simulink model "pipeadc_3b_model"  (R2024b)
settings: Solver=ode4  StartTime=0.0  StopTime=tstop  FixedStep=tstep  RelTol=1e-3
values from neighbouring files (symbols this model uses):
  amplitude = Vref    (= 1.5)    [pipeadc_3b.m]
  fsig = 1e3    (= 1000)    [pipeadc_3b.m]
  offset = 0    [pipeadc_3b.m]
  Vref = (Vrefp-Vrefn)    (= 1.5)    [pipeadc_3b.m]
libraries: simulink_extras x5
settings Model: Creator=koefinger  LastModifiedBy=koefinger

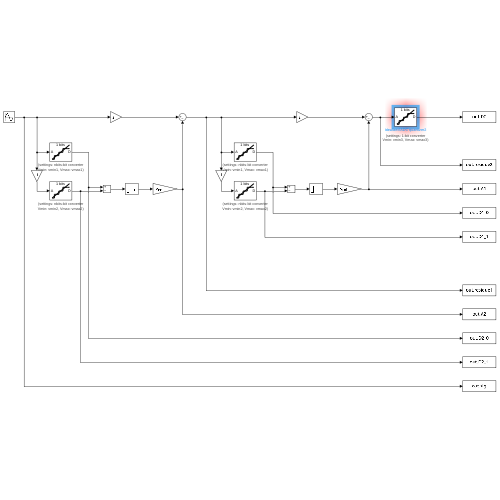
[thumbnail: Simulink's stored preview of the top-level diagram]
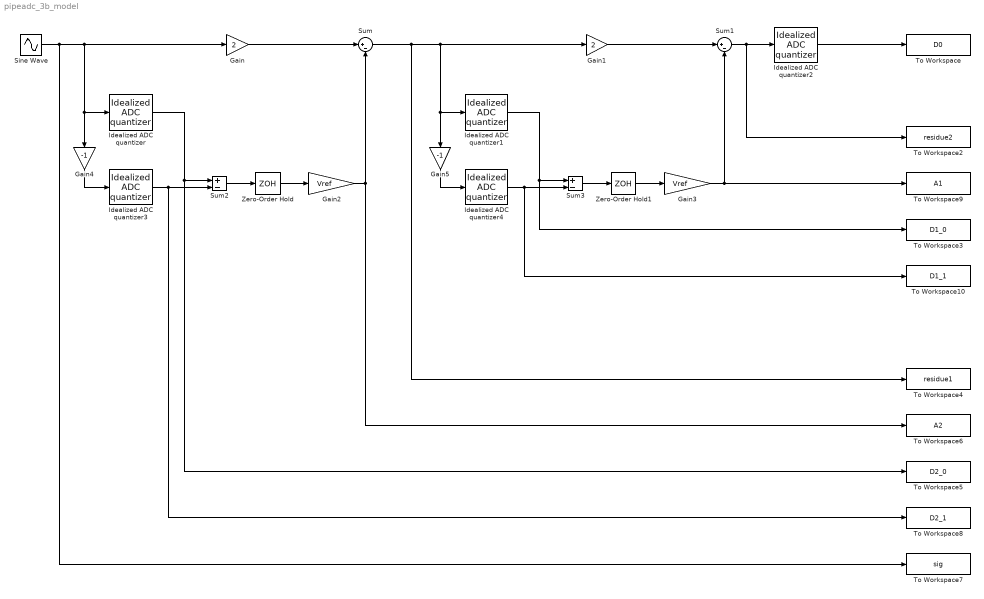
== system pipeadc_3b_model ==
  Gain : Gain  Gain=2
  Gain1 : Gain  Gain=2
  Gain2 : Gain  Gain=Vref
  Gain3 : Gain  Gain=Vref
  Gain4 : Gain  Gain=-1
  Gain5 : Gain  Gain=-1
  Idealized ADC quantizer : simulink_extras/Additional Discrete/Idealized ADC quantizer  NumberOfConverterBits=nbits  Vmin=vmin1  Vmax=vmax1  OutputDataType=int16  OutputNegativeValues=off
  Idealized ADC quantizer1 : simulink_extras/Additional Discrete/Idealized ADC quantizer  NumberOfConverterBits=nbits  Vmin=vmin1  Vmax=vmax1  OutputDataType=int16  OutputNegativeValues=off
  Idealized ADC quantizer2 : simulink_extras/Additional Discrete/Idealized ADC quantizer  NumberOfConverterBits=1  Vmin=vmin3  Vmax=vmax3  OutputDataType=int16  OutputNegativeValues=off
  Idealized ADC quantizer3 : simulink_extras/Additional Discrete/Idealized ADC quantizer  NumberOfConverterBits=nbits  Vmin=vmin2  Vmax=vmax2  OutputDataType=int16  OutputNegativeValues=off
  Idealized ADC quantizer4 : simulink_extras/Additional Discrete/Idealized ADC quantizer  NumberOfConverterBits=nbits  Vmin=vmin2  Vmax=vmax2  OutputDataType=int16  OutputNegativeValues=off
  Sine Wave : Sin  Amplitude=amplitude  Bias=offset  Frequency=2*pi*fsig  SampleTime=0
  Sum : Sum  Inputs=|+-
  Sum1 : Sum  Inputs=|+-
  Sum2 : Sum  Inputs=+-
  Sum3 : Sum  Inputs=+-
  To Workspace : ToWorkspace  VariableName=D0  SaveFormat=Timeseries  SampleTime=-1
  To Workspace10 : ToWorkspace  VariableName=D1_1  SaveFormat=Timeseries  SampleTime=-1
  To Workspace2 : ToWorkspace  VariableName=residue2  SaveFormat=Timeseries  SampleTime=-1
  To Workspace3 : ToWorkspace  VariableName=D1_0  SaveFormat=Timeseries  SampleTime=-1
  To Workspace4 : ToWorkspace  VariableName=residue1  SaveFormat=Timeseries  SampleTime=-1
  To Workspace5 : ToWorkspace  VariableName=D2_0  SaveFormat=Timeseries  SampleTime=-1
  To Workspace6 : ToWorkspace  VariableName=A2  SaveFormat=Timeseries  SampleTime=-1
  To Workspace7 : ToWorkspace  VariableName=sig  SaveFormat=Timeseries  SampleTime=-1
  To Workspace8 : ToWorkspace  VariableName=D2_1  SaveFormat=Timeseries  SampleTime=-1
  To Workspace9 : ToWorkspace  VariableName=A1  SaveFormat=Timeseries  SampleTime=-1
  Zero-Order Hold : ZeroOrderHold  SampleTime=-1
  Zero-Order Hold1 : ZeroOrderHold  SampleTime=-1
  wires:
  Sine Wave/1 -> To Workspace7/1, Gain4/1, Idealized ADC quantizer/1, Gain/1
  Zero-Order Hold/1 -> Gain2/1
  Gain/1 -> Sum/1
  Idealized ADC quantizer2/1 -> To Workspace/1
  Gain2/1 -> To Workspace6/1, Sum/2
  Idealized ADC quantizer3/1 -> To Workspace8/1, Sum2/2
  Idealized ADC quantizer/1 -> Sum2/1, To Workspace5/1
  Sum2/1 -> Zero-Order Hold/1
  Gain3/1 -> To Workspace9/1, Sum1/2
  Sum1/1 -> To Workspace2/1, Idealized ADC quantizer2/1
  Gain1/1 -> Sum1/1
  Idealized ADC quantizer4/1 -> To Workspace10/1, Sum3/2
  Sum3/1 -> Zero-Order Hold1/1
  Zero-Order Hold1/1 -> Gain3/1
  Sum/1 -> To Workspace4/1, Gain5/1, Idealized ADC quantizer1/1, Gain1/1
  Idealized ADC quantizer1/1 -> To Workspace3/1, Sum3/1
  Gain4/1 -> Idealized ADC quantizer3/1
  Gain5/1 -> Idealized ADC quantizer4/1
